simulink subsystem "TwoActuatorAWDSSC"  (R2025b)
settings: Solver=VariableStepAuto  StartTime=0.0  StopTime=10.0  RelTol=1e-3
undefined symbols (not defined in the file): DriveshftTrq1, DriveshftTrq2
libraries: fl_lib x5, nesl_utility_internal x2
settings Model: Creator=The MathWorks, Inc.  LastModifiedBy=The MathWorks, Inc.
settings OptimizationCC: ReuseModelBlockBuffer=off
settings RTWCC: GPUComputeCapability=3.5

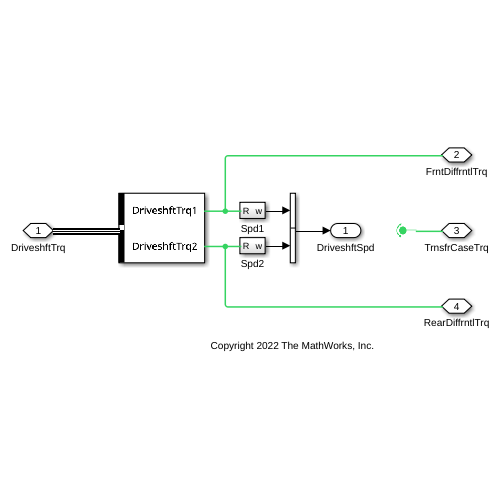
[thumbnail: Simulink's stored preview of the top-level diagram]
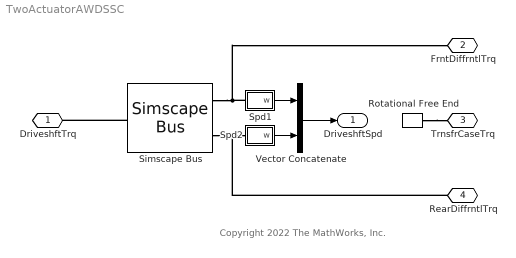
== system TwoActuatorAWDSSC ==
  note: Copyright 2022 The MathWorks, Inc.
  Rotational Free End : fl_lib/Mechanical/Rotational Elements/Rotational Free End  w_specify=off  w_priority=None  w=0 rad/s  w_nominal_specify=off  w_nominal_value=1  w_nominal_unit=rad/s
  Simscape Bus : SimscapeBus  HierarchyStrings=DriveshftTrq1;DriveshftTrq2
  Spd1 : Subsystem
  Spd2 : Subsystem
  Vector Concatenate : Concatenate
  DriveshftTrq : PMIOPort  Side=Left
  FrntDiffrntlTrq : PMIOPort  Port=2  Side=Right
  TrnsfrCaseTrq : PMIOPort  Port=3  Side=Right
  RearDiffrntlTrq : PMIOPort  Port=4  Side=Right
  DriveshftSpd : Outport  VectorParamsAs1DForOutWhenUnconnected=off
  wires:
  Spd2/1(w) -> Vector Concatenate/2
  Spd1/1(w) -> Vector Concatenate/1
  Vector Concatenate/1 -> DriveshftSpd/1
  connections:
  Simscape Bus/LConn1 -- Spd1/LConn1 -- FrntDiffrntlTrq/RConn1
  Simscape Bus/LConn2 -- Spd2/LConn1 -- RearDiffrntlTrq/RConn1
  Rotational Free End/LConn1 -- TrnsfrCaseTrq/RConn1
  Simscape Bus/RConn1 -- DriveshftTrq/RConn1

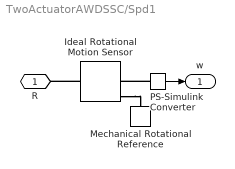
== system TwoActuatorAWDSSC/Spd1 ==
  Ideal Rotational Motion Sensor : fl_lib/Mechanical/Mechanical Sensors/Ideal Rotational Motion Sensor  reference=foundation.enum.MeasurementReference.difference  acceleration_port=false  velocity_port=true  position_port=true  wrap_angle=simscape.enum.onoff.off  offset=0 rad
  Mechanical Rotational Reference : fl_lib/Mechanical/Rotational Elements/Mechanical Rotational Reference
  PS-Simulink Converter : nesl_utility_internal/PS-Simulink Converter  PhysicalDomain=network_engine_domain  SubClassName=ps_output  LeftPortType=input  RightPortType=output  PseudoPeriodic=off  Frequencies=[]  VectorFormat=inherit  Unit=inherit  AffineConversion=off
  R : PMIOPort  Side=Left
  w : Outport
  wires:
  PS-Simulink Converter/1 -> w/1
  connections:
  PS-Simulink Converter/LConn1 -- Ideal Rotational Motion Sensor/RConn2
  Ideal Rotational Motion Sensor/LConn1 -- R/RConn1
  Ideal Rotational Motion Sensor/RConn1 -- Mechanical Rotational Reference/LConn1

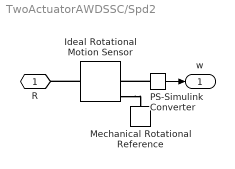
== system TwoActuatorAWDSSC/Spd2 ==
  Ideal Rotational Motion Sensor : fl_lib/Mechanical/Mechanical Sensors/Ideal Rotational Motion Sensor  reference=foundation.enum.MeasurementReference.difference  acceleration_port=false  velocity_port=true  position_port=true  wrap_angle=simscape.enum.onoff.off  offset=0 rad
  Mechanical Rotational Reference : fl_lib/Mechanical/Rotational Elements/Mechanical Rotational Reference
  PS-Simulink Converter : nesl_utility_internal/PS-Simulink Converter  PhysicalDomain=network_engine_domain  SubClassName=ps_output  LeftPortType=input  RightPortType=output  PseudoPeriodic=off  Frequencies=[]  VectorFormat=inherit  Unit=inherit  AffineConversion=off
  R : PMIOPort  Side=Left
  w : Outport
  wires:
  PS-Simulink Converter/1 -> w/1
  connections:
  Ideal Rotational Motion Sensor/RConn1 -- Mechanical Rotational Reference/LConn1
  Ideal Rotational Motion Sensor/LConn1 -- R/RConn1
  PS-Simulink Converter/LConn1 -- Ideal Rotational Motion Sensor/RConn2
